simulink model "youhua_1226"  (R2017b)
settings: Solver=ode1  StartTime=0.0  StopTime=Inf  FixedStep=0.0002  RelTol=1e-3
PreLoadFcn:
  | initFun_4P.m
PostLoadFcn:
  | , if any(exist('dsrtsu_mdlpostloadfcn', 'file') == [2, 3, 6]), try dsrtsu_mdlpostloadfcn('Execute', bdroot); catch fprintf('Error in PostLoadFcn (dsrtsu_mdlpostloadfcn) for model "%s":\n %s\n', bdroot, lasterr); end, end,
InitFcn:
  | initFun_4P
undefined symbols (not defined in the file): CMAES_B_initial, CMAES_C_initial, CMAES_chiN_initial, CMAES_counteval_initial, CMAES_D_initial, CMAES_eigeneval_initial, CMAES_invsqrtC_initial, CMAES_pc_initial, CMAES_ps_initial, CMAES_sigma_initial, CMAES_xmean_initial
libraries: rti1202lib_adc_class1 x20, simulink x8, dsparch4 x6, rti1202serlib x4, rti1202lib_dio_class1 x4, dsextras x3, rtiemclib x2, rti1202lib_dac_class1 x1, rtitasklib x1
(part 6 of 6)

== matlab function youhua_1226/CONTROL/Control and Display/OO/optimization ==
  data: oo_dtau_offset input; OOParamNo output; maxTorque input; optTrig input; optData input; metA input; param input; noParam input; optAlgo input; OOReset input; CMAES_xmean_initials input; CMAES_sigma_initial input; CMAES_D_initials input; CMAES_B_initials input; idx_prev input; initCheck_prev input; noDataPoints_prev input; ameba_state_prev input; surrogate_state_prev input; cmaes_state_prev input; CMAES_pc_prev input; CMAES_ps_prev input; CMAES_B_prev input; CMAES_D_prev input; CMAES_C_prev input; CMAES_invsqrtC_prev input; CMAES_eigeneval_prev input; CMAES_chiN_prev input; CMAES_sigma_prev input; CMAES_counteval_prev input; CMAES_xmean_prev input; optData_next output; param_next output; idx output; initCheck output; noDataPoints output; ameba_state output; surrogate_state output; cmaes_state output; CMAES_pc output; CMAES_ps output; CMAES_B output; CMAES_D output; CMAES_C output; CMAES_invsqrtC output; CMAES_eigeneval output; CMAES_chiN output; CMAES_sigma output; CMAES_counteval output; CMAES_xmean output; initDataSize output; current_param output; CMAES_weights output; X2 output
function [OOParamNo, optData_next, param_next, idx, initCheck, noDataPoints,...
    ameba_state, surrogate_state, cmaes_state,...
    CMAES_pc, CMAES_ps, CMAES_B, CMAES_D, CMAES_C, CMAES_invsqrtC,...
    CMAES_eigeneval, CMAES_chiN, CMAES_sigma, CMAES_counteval,...
    CMAES_xmean,...
    initDataSize, current_param, CMAES_weights, X2]= optFun(oo_dtau_offset,maxTorque,optTrig,optData,metA,...
    param, noParam, optAlgo,  OOReset,...
    CMAES_xmean_initials, CMAES_sigma_initial, CMAES_D_initials,...
    CMAES_B_initials,...
    idx_prev, initCheck_prev,noDataPoints_prev,...
    ameba_state_prev, surrogate_state_prev, cmaes_state_prev,...
    CMAES_pc_prev, CMAES_ps_prev, CMAES_B_prev, CMAES_D_prev,...
    CMAES_C_prev, CMAES_invsqrtC_prev,...
    CMAES_eigeneval_prev, CMAES_chiN_prev, CMAES_sigma_prev,...
    CMAES_counteval_prev,CMAES_xmean_prev)
  


param_next = param;
current_param = param;
idx = idx_prev;
optData_next = optData;
initCheck = initCheck_prev;
noDataPoints = noDataPoints_prev;
ameba_state = ameba_state_prev;
surrogate_state = surrogate_state_prev;
cmaes_state = cmaes_state_prev;




CMAES_pc = CMAES_pc_prev;
CMAES_ps = CMAES_ps_prev;
CMAES_B = CMAES_B_prev;
CMAES_D = CMAES_D_prev;
CMAES_C = CMAES_C_prev;
CMAES_invsqrtC = CMAES_invsqrtC_prev;
CMAES_eigeneval = CMAES_eigeneval_prev;
CMAES_chiN = CMAES_chiN_prev;
CMAES_sigma = CMAES_sigma_prev;
CMAES_counteval = CMAES_counteval_prev;
CMAES_xmean= CMAES_xmean_prev;
CMAES_weights = zeros(4, 1);
assert(noParam<5);
OOParamNo = noParam;

X2 = zeros(8, 4);

%%ameba parameters
alpha = 1;
gamma = 2;
rho = 0.5;
sigma = 0.5;

switch optAlgo
    case 1 % ameba
        initDataSize = noParam+1;
        genSize = 1;
    case 2 & 3 % surrogate based, 2: fifo; 3: all available data
        initDataSize = noParam*2+noParam*(noParam-1)+1;
        genSize = 1;
    case 4
        initDataSize = 4+floor(3*log(noParam));
        genSize = initDataSize;
        
    otherwise
        initDataSize = noParam+1;
        genSize =1;
end;


if OOReset == 1
    InitialParams = zeros(8, 5);
    %for step frequency
    
    
    initCheck = 0;
    idx = 0;
    noDataPoints = 0; % # of
    
    
    ameba_state = 0;
    surrogate_state = 0;
    cmaes_state = 0;
    
    
    
    CMAES_pc = zeros(4,1);
    CMAES_ps = zeros(4,1);
    CMAES_B = eye(4,4);
    CMAES_D = ones(4,1);
    CMAES_C = CMAES_B * diag(CMAES_D.^2) * CMAES_B';
    CMAES_invsqrtC = CMAES_B * diag(CMAES_D.^-1) * CMAES_B';
    CMAES_eigeneval = 0;
    
    
    CMAES_counteval = 0;
    %     CMAES_xmean= zeros(15,1);
    
    CMAES_chiN = noParam^0.5*(1-1/(4*noParam)+1/(21*noParam^2));
    
    %     [CMAES_sigma, CMAES_xmean]=reset_param(noParam);
    if isrow(CMAES_xmean_initials)
        CMAES_xmean = CMAES_xmean_initials';
    else
        CMAES_xmean = CMAES_xmean_initials;
    end;
    
    CMAES_sigma = CMAES_sigma_initial;
    CMAES_D = CMAES_D_initials;
     CMAES_B = [CMAES_B_initials(1:4)';CMAES_B_initials(5:8)';CMAES_B_initials(9:12)';CMAES_B_initials(13:16)'];
     % CMAES_invsqrtC=CMAES_invsqrtC_initial;%%%%%%%%%%%%%%%%%%%%%%%%%%%
    %         CMAES_xmean(1,1)=1.1;
    %     CMAES_sigma = 0.1;
    
    
    B = CMAES_B(1:noParam, 1:noParam);
    D = CMAES_D(1:noParam, 1);
    
    sigma  = CMAES_sigma;
    xmean = CMAES_xmean(1:noParam,1);
    
    
    assert(noParam<5)
    assert(initDataSize < 8);
    initx = zeros(noParam, initDataSize);
    
    switch optAlgo
        case 1
            
            for k=1:initDataSize,
                initx(:,k) = xmean + sigma * B * (D .* randn(noParam,1)); % m + sig * Normal(0,C)
                %                         x3(:,k) = xmean + sigma*C*randn(noParam,1); % m + sig * Normal(0,C)
                if noParam==4
                initx(:,k) = applyConstraints(initx(:,k), maxTorque, oo_dtau_offset);
                end;                
            end
            
        case 4     
            
            for k=1:initDataSize,
                initx(:,k) = xmean + sigma * B * (D .* randn(noParam,1)); % m + sig * Normal(0,C)
                %                         x3(:,k) = xmean + sigma*C*randn(noParam,1); % m + sig * Normal(0,C)
                if noParam==4
                initx(:,k) = applyConstraints(initx(:,k), maxTorque,oo_dtau_offset);
                end;
            end
            
            
        otherwise
    end;
    
    % constraint parameters
    
    initx(find(initx<0))=0;
    
    % sort parameters according to parameter 1, the peak desired torque,
    
    [~, iii] = sort(initx(1, :));
    initx = initx(:, iii);
    

    InitialParams(1:initDataSize,2:noParam+1) = initx';
    
  
    optData_next = InitialParams;
    param_next = zeros(size(param_next));
    param_next(1:noParam,1) = (optData_next(noDataPoints+1, 2:noParam+1))';
    
else
    
    %% update onlly when triggered
    if optTrig ==1
        idx = idx +1; % increase data point count
        
        if initCheck == 0 % initial data collection
            if idx<=initDataSize
                temp = optData;
                temp(idx, 2:noParam+1) = (param(1:noParam))';
                temp(idx, 1) = metA;
                optData_next = temp;
                %             noDataPoints = noDataPoints+1;
                param_next(1:noParam,1) = (optData(idx+1, 2:noParam+1))';
                %                 optData_next(end, 2:noParam+1) = param_next(1:noParam,1)';
                if idx == initDataSize
                    initCheck = 1;
                    ameba_state = 1;
                    surrogate_state = 1;
                    cmaes_state = 1;
                    idx = 0;
                end;
                
            end;
        end;
        
        
        if initCheck == 1
            
            switch optAlgo
                
                case 1 % ameba
                    
                    
                    noDataPoints = noParam+1; % # of points in memory
                    x = optData(1:noDataPoints,2:noParam+1); % all parameter values
                    y = optData(1:noDataPoints,1); % all cost function values
                    [y2, i2] = sort(y); % sort cost
                    x2 = x(i2, :); % parameter values in increasing order of cost
                    X2(1:noDataPoints, 1:noParam) = x2;
                    x0 = mean(x2(1:noDataPoints-1, :)); % centroid of all points exact the last one with highest y
                    xr = x0+alpha*(x0-x2(noDataPoints, :)); %reflected point
                    
                    switch ameba_state
                        
                        case 1 % first parameter point from optimization, the reflected point, new data already saved
                            
                            x(noDataPoints, :) = param(1:noParam,1)';
                            y(noDataPoints, 1) = metA;
                            
                            [y5, i5] = sort(y); % sort cost
                            x5 = x(i5, :); % parameter values in increasing order of cost
                            X2(1:noDataPoints, 1:noParam) = x5;
                            x05 = mean(x5(1:noDataPoints-1, :)); % centroid of all points exact the last one with highest y
                            xr5 = x05+alpha*(x05-x5(noDataPoints, :)); %reflected point
                            xr5(find(xr5<0))=0;
                            if noParam==4
                                temp_xr = applyConstraints(xr5', maxTorque, oo_dtau_offset);
                                xr5 = temp_xr';
                            end;
                            param_next(1:noParam,1) = xr5';
                            ameba_state = 2;
                        case 2 % compare new point with those in memory, noDataPoints count of data point in memory, and 1 new data point
                            if metA>=y2(1) && metA<y2(noDataPoints-1)
                                y2(noDataPoints,1) = metA;
                                x2(noDataPoints, :) = param(1:noParam,1)';
                                ameba_state = 2;
                                %                             tempx = (optData_next(1:noDataPoints,2:noParam+1))';
                                %                             tempy = (optData_next(1:noDataPoints,1))' ;
                                %                             tempx0 = zeros(size(tempx(:,1)));
                                [y3, i3] = sort(y2);
                                x3 = x2(i3, :);
                                
                                x02= mean(x3(1:noDataPoints-1, :));
                                
                                xr2 = x02+alpha*(x02-x3(noDataPoints, :));
                                xr2(find(xr2<0))=0;
                                if noParam==4
                                    temp_xr = applyConstraints(xr2', maxTorque, oo_dtau_offset);
                                    xr2 = temp_xr';
                                end;
                                param_next(1:noParam, 1) = xr2';
                                
                            elseif metA<y2(1)
                                xe = x0+gamma*(xr-x0);
                                xe(find(xe<0))=0;
                                if noParam==4
                                    temp_xr = applyConstraints(xe', maxTorque, oo_dtau_offset);
                                    xe = temp_xr';
                                end;
                                param_next(1:noParam, 1) = xe';
                                ameba_state = 3;
                                
                                % temp saving of reflected data point in memory
                                optData_next(noDataPoints+1, 2:noParam+1) = param(1:noParam,1)';
                                optData_next(noDataPoints+1, 1) = metA;
                            else % f(xr)>=f(x_n)
                                if metA>=y2(noDataPoints, 1)
                                    xc = x0+rho*(x2(noDataPoints,:)-x0);
                                else
                                    xc = x0+rho*(xr-x0);
                                end
                                xc(find(xc<0))=0;
                                if noParam==4
                                    temp_xr = applyConstraints(xc', maxTorque, oo_dtau_offset);
                                    xc = temp_xr';
                                end;
                                param_next(1:noParam,1) = xc';
                                ameba_state = 4;
                            end;
                            
                            optData_next(1:noDataPoints, 2:noParam+1) = x2;
                            optData_next(1:noDataPoints, 1) = y2;
                            %                             optData_next(end, 2:noParam+1) = param_next(1:noParam, 1)';
                            
                        case 3 % expanded point evaluated
                            if metA<optData(noDataPoints+1, 1)
                                y2(noDataPoints,1) = metA;
                                x2(noDataPoints, :) = param(1:noParam,1)'; %%% not working
                                
                            else
                                y2(noDataPoints,1) = optData(noDataPoints+1, 1);
                                x2(noDataPoints, :) = optData(noDataPoints+1, 2:noParam+1);
                                
                            end;
                            
                            optData_next(1:noDataPoints, 2:noParam+1) = x2;
                            optData_next(1:noDataPoints, 1) = y2;
                            
                            
                            [y3, i3] = sort(y2);
                            x3 = x2(i3, :);
                            
                            x02= mean(x3(1:noDataPoints-1, :));
                            
                            xr2 = x02+alpha*(x02-x3(noDataPoints,:));
                            xr2(find(xr2<0))=0;
                            if noParam==4
                                temp_xr = applyConstraints(xr2', maxTorque, oo_dtau_offset);
                                xr2 = temp_xr';
                            end;
                            param_next(1:noParam, 1) = xr2';
                            ameba_state = 2;
                            %                             optData_next(end, 2:noParam+1) = param_next(1:noParam, 1)';
                        case 4
                            if metA<y2(noDataPoints,1)
                                
                                y2(noDataPoints,1) = metA;
                                x2(noDataPoints, :) = param(1:noParam,1)';
                                optData_next(1:noDataPoints, 2:noParam+1) = x2;
                                optData_next(1:noDataPoints, 1) = y2;
                                
                                
                                [y3, i3] = sort(y2);
                                x3 = x2(i3,:);
                                
                                x02= mean(x3(1:noDataPoints-1, :));
                                
                                xr2 = x02+alpha*(x02-x3(noDataPoints, :));
                                xr2(find(xr2<0))=0;
                                if noParam==4
                                    temp_xr = applyConstraints(xr2', maxTorque, oo_dtau_offset);
                                    xr2 = temp_xr';
                                end;
                                param_next(1:noParam, 1) = xr2';
                                ameba_state = 2;
                            else
                                for i=2:1:(noParam+1)
                                    x2(i,:)= x2(1,:)+sigma*(x2(i,:)-x2(1,:));
                                    if noParam ==4
                                    temp_xr=applyConstraints(x2(i,:)', maxTorque, oo_dtau_offset);
                                    x2(i,:) = temp_xr';
                                    end;

                                end;
                                x2(find(x2<0))=0;

                                optData_next(1:noDataPoints,2:noParam+1) = x2;
                                optData_next(1:noDataPoints, 1) = y2;
                                
                                noDataPoints = 1;
                                initCheck = 0;
                                ameba_state = 0;
                                
                                surrogate_state = 0;
                                cmaes_state = 0;
                                idx = 1;
                                param_next(1:noParam,1) = x2(2, :)';
                            end;
                            %                             optData_next(end, 2:noParam+1) = param_next(1:noParam, 1)';
                        otherwise
                    end;
                case 2
                    %                 x3 = x2;
                    %                 y3 = y2;
                    %                 polyfit(x2(1,:), y2, 2);
                    
                case 3
                    %                 switch surrogate_state
                    %                     case 1
                    %                     case 2
                    %                     case 3
                    %                     otherwise
                    %                 end;
                case 4
                    
                    
                    
                    noDataPoints = initDataSize; % # of points in memory
                    x = optData(1:noDataPoints,2:noParam+1); % all parameter values
                    y = optData(1:noDataPoints,1); % all cost function values
                    x(noDataPoints, :) = param(1:noParam,1)';
                    y(noDataPoints, 1) = metA;
                    
                    [y2, i2] = sort(y); % sort cost
                    x2 = x(i2, :); % parameter values in increasing order of cost
                    X2(1:noDataPoints, 1:noParam) = x2;
                    x22 = x2'; %x in column
                    lambda = initDataSize;
                    assert(lambda<=8);
                    mu=lambda/2;
                    
                    
                    temp_w = zeros(4,1);
                    mu = floor(mu);
                    for j=1:1:mu
                        temp_w(j) = log(mu+1/2)-log(j);
                    end
                    
                    weights = temp_w(1:mu)/sum(temp_w(1:mu));
                    CMAES_weights(1:mu,1) = weights;
                    
                    mueff = sum(weights)^2/sum(weights.^2);
                    
                    cc = (4+mueff/noParam)/(noParam+4+2*mueff/noParam);
                    cs = (mueff+2) / (noParam+mueff+5);
                    c1 = 2 / ((noParam+1.3)^2+mueff);
                    cmu=min(1-c1, 2*(mueff-2+1/mueff)/((noParam+2)^2+mueff));
                    damps = 1 + 2*max(0, sqrt((mueff-1)/(noParam+1))-1)+cs;
                    
                    pc = CMAES_pc(1:noParam, 1);
                    ps = CMAES_ps(1:noParam, 1);
                    %                     B = zeros(noParam, noParam);
                    %                     D = zeros(noParam, 1);
                    %                     C = zeros(noParam, noParam);
                    B = CMAES_B(1:noParam, 1:noParam);
                    D = CMAES_D(1:noParam, 1);
                    C = CMAES_C(1:noParam, 1:noParam);
                    eigeneval = CMAES_eigeneval;
                    chiN =CMAES_chiN;
                    sigma  = CMAES_sigma;
                    counteval = CMAES_counteval;
                    xold = CMAES_xmean(1:noParam,1);
                    invsqrtC = CMAES_invsqrtC(1:noParam, 1:noParam);
                    
                    counteval = counteval+lambda;
%                     xold  = xmean;
                    %updates;
                    
                    xmean = zeros(noParam, 1);
                    for h=1:1:noParam
                        xmean(h, 1) = x22(h, 1:mu)*weights;
                    end;
                    
%                     xmean = x22(:, 1:mu)*weights;
                    
                    
                    
                    ps = (1-cs)*ps ...
                        + sqrt(cs*(2-cs)*mueff) * invsqrtC * (xmean-xold) / sigma;
                    hsig = norm(ps)/sqrt(1-(1-cs)^(2*counteval/lambda))/chiN < 1.4 + 2/(noParam+1);
                    pc = (1-cc)*pc ...
                        + hsig * sqrt(cc*(2-cc)*mueff) * (xmean-xold) / sigma;
                    
                    %                     assert(mu<20);
                    artmp = (1/sigma) * (x22(:,1:mu)-repmat(xold,1,mu));
                    C = (1-c1-cmu) * C ...                  % regard old matrix
                        + c1 * (pc*pc' ...                 % plus rank one update
                        + (1-hsig) * cc*(2-cc) * C) ... % minor correction if hsig==0
                        + cmu * artmp * diag(weights) * artmp'; % plus rank mu update
                    
                    % Adapt step size sigma
                    sigma = sigma * exp((cs/damps)*(norm(ps)/chiN - 1));
                    if counteval - eigeneval > lambda/(c1+cmu)/noParam/10  % to achieve O(N^2)
                        eigeneval = counteval;
                        C_tmp = triu(C) + triu(C,1)'; % enforce symmetry
                        [B,D_tmp] = eig(C_tmp);           % eigen decomposition, B==normalized eigenvectors
                        
                        D = sqrt(diag(D_tmp));        % D is a vector of standard deviations now
                        B = real(B);
                        D = real(D);
                        invsqrtC = B * diag(D.^-1) * B'; % to be fixed
                    end
                    
                    
                    CMAES_pc(1:noParam, 1) = pc;
                    CMAES_ps(1:noParam, 1) = ps;
                    CMAES_B(1:noParam, 1:noParam) = B; % to be fixed
                    CMAES_D(1:noParam, 1)=D(1:noParam, 1);% to be fixed
                    CMAES_C(1:noParam, 1:noParam)=C;
                    CMAES_eigeneval=eigeneval;
                    CMAES_chiN=chiN;
                    CMAES_sigma=sigma;
                    CMAES_counteval=counteval;
                    CMAES_xmean(1:noParam,1)=xmean;
                    CMAES_invsqrtC(1:noParam, 1:noParam) =invsqrtC;
                    
                    
                    initCheck = 0;
                    
                    
                    
                    x3 = zeros(noParam, lambda);
                    for k=1:lambda,
                        x3(:,k) = xmean + sigma * B * (D .* randn(noParam,1)); % m + sig * Normal(0,C)
                        if noParam == 4
                            temp_xr= applyConstraints(x3(:,k), maxTorque, oo_dtau_offset);
                            x3(:,k) = temp_xr;
                        end;
                        %                         x3(:,k) = xmean + sigma*C*randn(noParam,1); % m + sig * Normal(0,C)
                    end
                    %%
                    
                    x3(find(x3<0))=0;
                    

                    % sort parameters according to parameter 1, the peak desired torque,
                    
                    [~, iii] = sort(x3(1, :));
                    x3 = x3(:, iii);
                    %%
                    
                    optData_next(1:noDataPoints,2:noParam+1) = x3';
                    optData_next(1:noDataPoints,1) = zeros(noDataPoints,1);
                    
                    param_next(1:noParam) = x3(:,1);
                    
                    %                 switch cmaes_state
                    %                     case 1
                    %                     case 2
                    %                     case 3
                    %                     otherwise
                    %                 end;
                otherwise
            end;
        end;
        
    end;
end;
return;


function params = applyConstraints(original_params, maxTorque, oo_dtau_offset)
params = zeros(length(original_params), 1);

% assert params to be column vector;
if iscolumn(original_params)
    params = original_params;
else
    params = original_params';
end;


params(find(params<0))=0;
params(3,1) = max(10, params(3,1)); % rise time at least 10%
params(4,1) = max(10, params(4,1)); % drop time at least 5%
params(4,1) = min(40, params(4,1)); % drop time at most 20%
params(3,1) = min(40, params(3,1)); % drop time at most 20%

%% max peak desired torque 100Nm
params(1,1) = min(maxTorque-oo_dtau_offset, params(1,1));

peakTorque = params(1,1)+oo_dtau_offset;
if peakTorque < 0.75*maxTorque
    maxParam2 = 110;
else
    maxParam2 = 110-10*(peakTorque-0.75*maxTorque)/(0.25*maxTorque);
end;

params(2,1) = min(maxParam2, max(20,params(2,1)));

%% max peak 
% if params(2,1)/2>60
%     params(2,1)=120;
% end;
% if peak time + drop time go beyong 65%stride, shorten drop time; then
% lower limit 
if params(4,1)/2+params(2,1)/2>65
%     params(2,1)=2*(65-params(4,1)/2);
    params(4,1) = max(2*(65-params(2,1)/2),10);
end;
% if torque starts too early, reduce rise time
if params(2,1)/2-params(3,1)<5
    params(3,1) = max(params(2,1)/2-5, 10);
%     params(2,1)=2*(params(3,1)+5);
end;


return;

== matlab function youhua_1226/CONTROL/Control and Display/learning data write/filtered step data write/MATLAB Function2 ==
  data: bt_reset3 input; indices input; filtered_step_data input; filtered_step_data_in input; filtered_step_data_out output; learningMode input
function filtered_step_data_out = fcn(bt_reset3, indices, filtered_step_data, filtered_step_data_in, learningMode)
%#codegen
time_index = indices(1);
ankle_index = indices(2);
switch learningMode
    case 0 
        i = ankle_index;
    case 1
        i = time_index;
    otherwise
        i = time_index;
end
if (bt_reset3==1)
    filtered_step_data_out = zeros(size(filtered_step_data_in));
% else if time_index ==1
%         filtered_step_data_out = filtered_step_data_in;
%         [b, a] = butter(3, 0.2, 'low');
%         filtered_step_data_out(2, :) = filter(b, a, filtered_step_data_in(2,:));
    else
        filtered_step_data_out = filtered_step_data_in;
%     end
filtered_step_data_out(1, i) = filtered_step_data(3); % torque error
filtered_step_data_out(2, i) = filtered_step_data(2); % learned position
        
end;

== matlab function youhua_1226/CONTROL/Control and Display/learning data read/filtered step data read/Step Data Access ==
  data: oldD output; indices input; oldSD input; CommDelayCycle input; learningMode input
 function oldD = fcn2(indices, oldSD, CommDelayCycle, learningMode)
%#eml

time_index = indices(1);
ankle_index = indices(2);
switch learningMode
    case 0 
        i = ankle_index;
    case 1
        i = time_index;
    otherwise
        i = time_index;
end

oldD = zeros(3,1);
oldD(1) = oldSD(1, i);
oldD(2)= oldSD(2, i);
oldD(3) = oldSD(2, i+CommDelayCycle);
return

== matlab function youhua_1226/CONTROL/Control and Display/OODataGroupin ==
  data: metA input; optdata output; paramNo input; param input
function optdata = fcn(metA, paramNo, param)

optdata = zeros(6, 1);
optdata(1,1) = metA;
optdata(2,1) = paramNo;
optdata(3:end,1) = param;
